simulink model "FwModelDirectWay"  (R2022b)
settings: Solver=FixedStepDiscrete  StartTime=0.0  StopTime=1  FixedStep=1e-6  RelTol=1e-3
values from neighbouring files (symbols this model uses):
  Ts = 0.0001    [Motor_PIParam_Get2.m]
undefined symbols (not defined in the file or in its folder): DiscIntNeverNeededParam, Motor_flux, Motor_Ld_Indctances, Motor_Lq_Indctances, Motor_Pn, Motor_Rs
libraries: powerlib_extras x2, spsGroundLib x1, spsPermanentMagnetSynchronousMachineLib x1, spsThreePhaseVIMeasurementLib x1, spsUniversalBridgeLib x1, spsDCVoltageSourceLib x1, spspowerguiLib x1
settings Model: DataDictionary=modelDictionary.sldd  Creator=yll  LastModifiedBy=yll

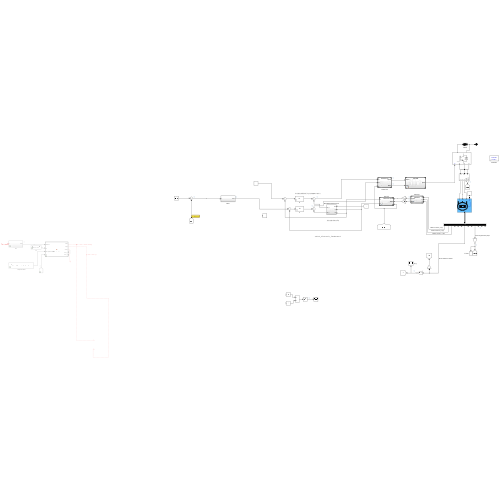
[thumbnail: Simulink's stored preview of the top-level diagram]
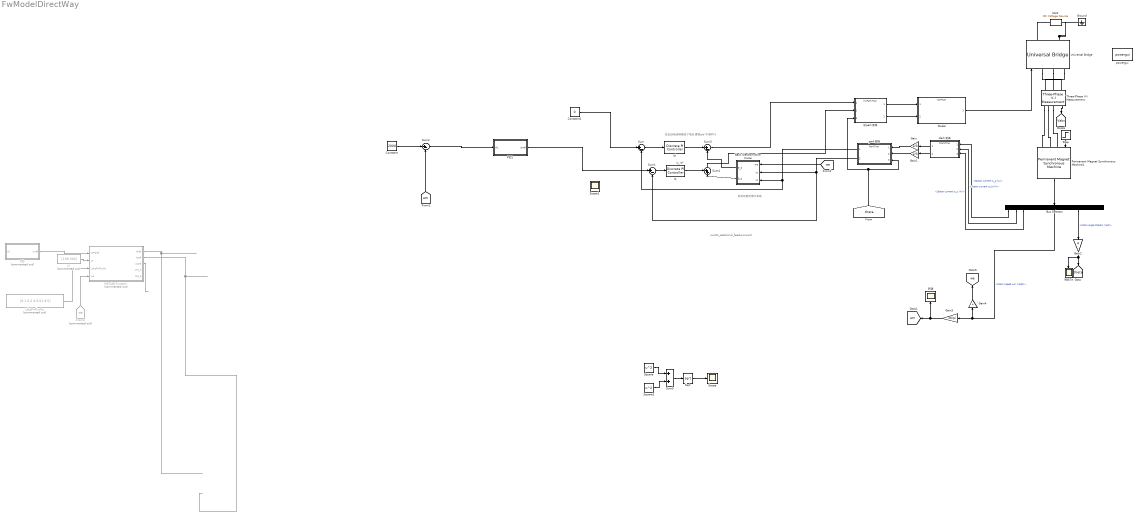
== system FwModelDirectWay ==
  note: switch_electronic_feedworward
  note: iq_ref
  note: 反电动势反馈子系统
  note: 在此处电流转换成了电压,要调pid 不调不行
  Back Electromotive Force : Subsystem
  Bus Selector : BusSelector  OutputSignals=Stator current is_a (A),Stator current is_b (A),Stator current is_c (A),Hall effect signal h_a,Hall effect signal h_b,Hall effect signal h_c,Rotor speed wm (rad/s),Stator current is_q (A),Stator current is_d (A),Rotor angle thetam (rad),Electromagnetic torque Te (N*m),Stator current is_q (A),Stator current is_d (A)
  Constant : Constant  Value=2000
  Constant1 : Constant  Value=0
  From3 : From  Commented=on  GotoTag=we  TagVisibility=global
  Gain : Gain  Gain=2/3
  Gain1 : Gain  Gain=2/3
  Gain2 : Gain  Gain=4
  Gain3 : Gain  Gain=30/pi
  Gain4 : Gain  Gain=4
  Ground : spsGroundLib/Ground  LConnTagsString=a
  Id : powerlib_extras/Discrete  Control Blocks/Discrete PI Controller  Kp=50  Ki=250  Par_Limits=[4000 -4000]  Init=0  Ts=1e-6
  Iq : powerlib_extras/Discrete  Control Blocks/Discrete PI Controller  Kp=50  Ki=250  Par_Limits=[4000 -4000]  Init=0  Ts=1e-6
  LdLqPnFluxRs : Constant  Commented=on  Value=[0.1 0.2 4 0.01 9.5]
  MATLAB Function : MATLAB Function  Commented=on  TreatAsAtomicUnit=on
  Model : ModelReference  ModelNameDialog=SVPWM.slx  SimulationMode=Normal  ModelReferenceVersion=1.6
  PID : Subsystem  Commented=on  VariantControl=true
  PID1 : Subsystem  VariantControl=true
  Permanent Magnet Synchronous Machine1 : spsPermanentMagnetSynchronousMachineLib/Permanent Magnet Synchronous Machine  NbPhases=3  FluxDistribution=Sinusoidal  RotorType=Salient-pole  MechanicalLoad=Torque Tm  PresetModel=No  ShowDetailedParameters=on  MeasurementBus=off  Resistance=Motor_Rs  Inductance=8.5e-3  dqInductances=[Motor_Ld_Indctances Motor_Lq_Indctances]  La=Motor_Ld_Indctances  MachineConstant=Flux linkage established by magnets (V.s)  Flux=Motor_flux  VoltageCst=145.1039  TorqueCst=1.2  Flat=120  Mechanical=[0.003 0 Motor_Pn 0]  PolePairs=2  InitialConditions=[0,0, 0,0]  InitialConditions5ph=[0 0 0 0 0 0]  RefAngle=Aligned with phase A axis (original Park)  IterativeDiscreteModel=Trapezoidal robust  TsBlock=-1  TsPowergui=0
  Scope : Scope
  Scope1 : Scope
  Sqrt : Sqrt
  Square : Math  Operator=square
  Square1 : Math  Operator=square
  Step : Step  Time=0.6  After=2  SampleTime=0
  Sum{,1..3} (4 alike) : Sum  Inputs=|+-
  Sum4 : Sum  Inputs=++|
  Sum5 : Sum
  Three-Phase V-I Measurement : spsThreePhaseVIMeasurementLib/Three-Phase V-I Measurement  VoltageMeasurement=phase-to-ground  SetLabelV=off  LabelV=Vabc  Vpu=off  VpuLL=off  CurrentMeasurement=yes  SetLabelI=off  LabelI=Iabc  Ipu=off  Pbase=100e6  Vbase=500e3  OutputType=Complex  PhasorSimulation=off  PSBequivalent=0
  UI : Constant  Commented=on  Value=[138 300]
  Universal Bridge : spsUniversalBridgeLib/Universal Bridge  Arms=3  SnubberResistance=1e3  SnubberCapacitance=inf  Device=IGBT / Diodes  Ron=1e-6  Lon=0  ForwardVoltages="[  0  0  ]"  ForwardVoltage="[  0  0  ]"  GTOparameters=[ 10e-6 , 20e-6 ]  IGBTparameters=[ 1e-6 , 2e-6 ]  Measurements=None  Measurements_2=None  converterType=Rectifier
  Vdc2 : spsDCVoltageSourceLib/DC Voltage Source  Amplitude=240  Measurements=None
  clark变换 : ModelReference  ModelNameDialog=ClarkTran.slx  SimulationMode=Normal  ModelReferenceVersion=1.13
  park变换 : ModelReference  ModelNameDialog=ParkTran.slx  SimulationMode=Normal  ModelReferenceVersion=1.9
  powergui : spspowerguiLib/powergui  Priority=1  SimulationMode=Discrete  SampleTime=1e-6  frequency=60  Iterations=50  frequencyindice=0  Pbase=100e6  ErrMax=1e-4  UnitsV=kV  UnitsW=MW  buscounter=0  FunctionMessages=off  echomessages=off  EnableUseOfTLC=off  CurrentSourceSwitches=off  DisableSnubberDevices=off  DisableRonSwitches=off  DisableVfSwitches=off  DisplayEquations=off  AutomaticDiscreteSolvers=off  SolverType=Tustin/Backward Euler (TBE)  Interpol=off  ExternalGateDelay=off  methode=off  Ts=10  x0status=blocks  SPID=off  SwTol=0  HookPort=off  NonlinearTolerance=1e-4  nMaxIteration=100  ContinueOnMaxIteration=off  RestoreLinks=warning  ResistiveCurrentMeasurement=off  Frange=[0:2:500]  Ylog=off  Xlog=on  ShowGrid=off  save=off  variable=ZData  structure=current_abc  ZoomFFT=off  StartTime=0.1  cycles=1  DisplayStyle=1  fundamental=1  FreqAxis=off  MaxFrequency=100  frequencyindicesteady=1  RmsSteady=1  display=off
  转矩Te : Scope
  转速 : Scope
  逆park变换 : ModelReference  ModelNameDialog=InvParkTran.slx  SimulationMode=Normal  ModelReferenceVersion=1.8
  tag scope: Vabc=global, theta=global, we=global, wm=global
  wires:
  Step/1 -> Permanent Magnet Synchronous Machine1/1
  Three-Phase V-I Measurement/1 -> [Vabc]
  Model/1 -> Universal Bridge/1
  Iq/1 -> Sum4/1
  Square1/1 -> Sum5/2
  clark变换/1 -> Gain/1
  Gain/1 -> park变换/1
  Back Electromotive Force/2(E_q) -> Sum4/2
  Square/1 -> Sum5/1
  [wm] -> Sum2/2
  Back Electromotive Force/1(E_d) -> Sum3/2
  Sum5/1 -> Sqrt/1
  [theta] -> 逆park变换/3, park变换/3
  clark变换/2 -> Gain1/1
  [we] -> Back Electromotive Force/1(we)
  park变换/1 -> Sum/2, Back Electromotive Force/3(id)
  Id/1 -> Sum3/1
  Sqrt/1 -> Scope/1
  Gain1/1 -> park变换/2
  Bus Selector/3 -> clark变换/3  "<Stator current is_c (A)>"
  逆park变换/2 -> Model/2
  Sum/1 -> Id/1
  Sum3/1 -> 逆park变换/1
  Sum4/1 -> 逆park变换/2
  逆park变换/1 -> Model/1
  park变换/2 -> Sum1/2, Back Electromotive Force/2(iq)
  Sum1/1 -> Iq/1
  Bus Selector/1 -> clark变换/1  "<Stator current is_a (A)>"
  Permanent Magnet Synchronous Machine1/1 -> Bus Selector/1
  Bus Selector/2 -> clark变换/2  "<Stator current is_b (A)>"
  Gain2/1 -> 转矩Te/1, [theta]
  Bus Selector/10 -> Gain2/1  "<Rotor angle thetam (rad)>"
  Gain4/1 -> [we]
  Gain3/1 -> [wm], 转速/1
  Bus Selector/7 -> Gain3/1, Gain4/1  "<Rotor speed wm (rad/s)>"
  Constant/1 -> Sum2/1
  From3/1 -> MATLAB Function/4(we)
  LdLqPnFluxRs/1 -> MATLAB Function/3(LdLqPnFluxRs)
  MATLAB Function/1(idref) -> ?
  UI/1 -> MATLAB Function/2(UI)
  PID/1(isref) -> MATLAB Function/1(isPidref)
  MATLAB Function/2(iqref) -> ?
  MATLAB Function/3(Zone) -> ?
  ? -> PID/1(In1)
  Sum2/1 -> PID1/1(In1)
  Constant1/1 -> Sum/1
  PID1/1(isref) -> Sum1/1
  connections:
  Universal Bridge/RConn2 -- Ground/LConn1 -- Vdc2/LConn1
  Vdc2/RConn1 -- Universal Bridge/RConn1
  Three-Phase V-I Measurement/RConn1 -- Permanent Magnet Synchronous Machine1/LConn1
  Three-Phase V-I Measurement/RConn3 -- Permanent Magnet Synchronous Machine1/LConn3
  Universal Bridge/LConn3 -- Three-Phase V-I Measurement/LConn3
  Three-Phase V-I Measurement/RConn2 -- Permanent Magnet Synchronous Machine1/LConn2
  Universal Bridge/LConn1 -- Three-Phase V-I Measurement/LConn1
  Universal Bridge/LConn2 -- Three-Phase V-I Measurement/LConn2

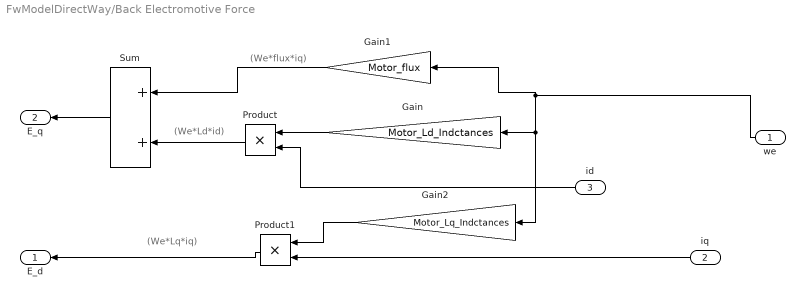
== system FwModelDirectWay/Back Electromotive Force ==
  note: (We*Lq*iq)
  note: (We*flux*iq)
  note: (We*Ld*id)
  we : Inport
  iq : Inport  Port=2
  id : Inport  Port=3
  Gain : Gain  Gain=Motor_Ld_Indctances
  Gain1 : Gain  Gain=Motor_flux
  Gain2 : Gain  Gain=Motor_Lq_Indctances
  Product : Product
  Product1 : Product
  Sum : Sum
  E_d : Outport
  E_q : Outport  Port=2
  wires:
  we/1 -> Gain2/1, Gain/1, Gain1/1
  Product1/1 -> E_d/1
  Gain1/1 -> Sum/1
  Sum/1 -> E_q/1
  Product/1 -> Sum/2
  id/1 -> Product/2
  iq/1 -> Product1/2
  Gain2/1 -> Product1/1
  Gain/1 -> Product/1

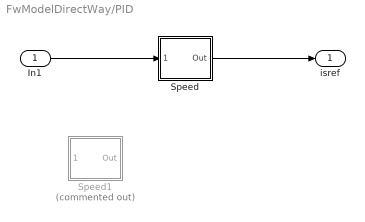
== system FwModelDirectWay/PID ==
  In1 : Inport
  Speed : Subsystem  AncestorBlock=|  DialogController=POWERSYS.PowerSysDialog  mask(Discrete PI Controller){Kpw=1, Kiw=1*50, Ba=0, Par_Limits=[3000 -3000], Init=0, Ts=1e-6}
      | powerlib_extras/Discrete 
      | Control Blocks/Discrete
      | PI Controller
      mask prompts: Kpw "Proportional gain (Kp):"; Kiw "Integral gain (Ki):"; Ba "feedback gain (Ba)"; Par_Limits "Output limits: [ Upper   Lower ]"; Init "Output initial value:"; Ts "Sample time:"
      mask help: This block implements a discrete PI controller.
      mask init:
      | UpperLimit=Par_Limits(1);
      | LowerLimit=Par_Limits(2);
      | power_initmask();
      settings: LibrarySourceBlock=|
      | powerlib_extras/Discrete
      | Control Blocks/Discrete
      | PI Controller
      mask Help: This block is part of a subset of blocks in the Extras library that does not have documentation associated with it, other than the block mask description.
      mask Display: disp('PI');
  Speed1 : Subsystem  Commented=on  AncestorBlock=|  DialogController=POWERSYS.PowerSysDialog  mask(Discrete PI Controller){Kpw=0.14, Kiw=0.14*50, Ba=0, Par_Limits=[800 -800], Init=0, Ts=Ts}
      | powerlib_extras/Discrete 
      | Control Blocks/Discrete
      | PI Controller
      mask prompts: Kpw "Proportional gain (Kp):"; Kiw "Integral gain (Ki):"; Ba "feedback gain (Ba)"; Par_Limits "Output limits: [ Upper   Lower ]"; Init "Output initial value:"; Ts "Sample time:"
      mask help: This block implements a discrete PI controller.
      mask init:
      | UpperLimit=Par_Limits(1);
      | LowerLimit=Par_Limits(2);
      | power_initmask();
      settings: LibrarySourceBlock=|
      | powerlib_extras/Discrete
      | Control Blocks/Discrete
      | PI Controller
      mask Help: This block is part of a subset of blocks in the Extras library that does not have documentation associated with it, other than the block mask description.
      mask Display: disp('PI');
  isref : Outport
  wires:
  Speed/1(Out) -> isref/1
  In1/1 -> Speed/1(Error)

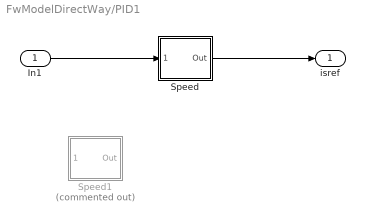
== system FwModelDirectWay/PID1 ==
  In1 : Inport
  Speed : Subsystem  AncestorBlock=|  DialogController=POWERSYS.PowerSysDialog  mask(Discrete PI Controller){Kpw=0.14, Kiw=0.14*50, Ba=0, Par_Limits=[6000 -6000], Init=0, Ts=1e-6}
      | powerlib_extras/Discrete 
      | Control Blocks/Discrete
      | PI Controller
      mask prompts: Kpw "Proportional gain (Kp):"; Kiw "Integral gain (Ki):"; Ba "feedback gain (Ba)"; Par_Limits "Output limits: [ Upper   Lower ]"; Init "Output initial value:"; Ts "Sample time:"
      mask help: This block implements a discrete PI controller.
      mask init:
      | UpperLimit=Par_Limits(1);
      | LowerLimit=Par_Limits(2);
      | power_initmask();
      settings: LibrarySourceBlock=|
      | powerlib_extras/Discrete
      | Control Blocks/Discrete
      | PI Controller
      mask Help: This block is part of a subset of blocks in the Extras library that does not have documentation associated with it, other than the block mask description.
      mask Display: disp('PI');
  Speed1 : Subsystem  Commented=on  AncestorBlock=|  DialogController=POWERSYS.PowerSysDialog  mask(Discrete PI Controller){Kpw=0.14, Kiw=0.14*50, Ba=0, Par_Limits=[800 -800], Init=0, Ts=Ts}
      | powerlib_extras/Discrete 
      | Control Blocks/Discrete
      | PI Controller
      mask prompts: Kpw "Proportional gain (Kp):"; Kiw "Integral gain (Ki):"; Ba "feedback gain (Ba)"; Par_Limits "Output limits: [ Upper   Lower ]"; Init "Output initial value:"; Ts "Sample time:"
      mask help: This block implements a discrete PI controller.
      mask init:
      | UpperLimit=Par_Limits(1);
      | LowerLimit=Par_Limits(2);
      | power_initmask();
      settings: LibrarySourceBlock=|
      | powerlib_extras/Discrete
      | Control Blocks/Discrete
      | PI Controller
      mask Help: This block is part of a subset of blocks in the Extras library that does not have documentation associated with it, other than the block mask description.
      mask Display: disp('PI');
  isref : Outport
  wires:
  Speed/1(Out) -> isref/1
  In1/1 -> Speed/1(Error)

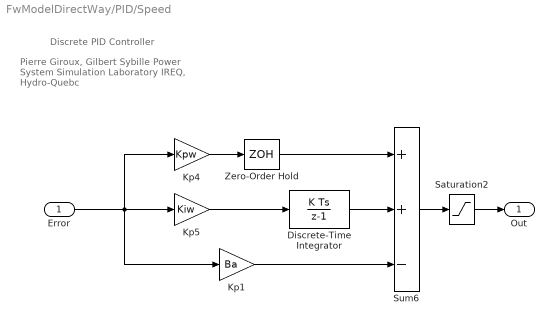
== system FwModelDirectWay/PID/Speed ==
  note: Pierre Giroux, Gilbert Sybille
      | Power System Simulation Laboratory
      | IREQ, Hydro-Quebc
  note: Discrete PID Controller
  Error : Inport  SampleTime=Ts
  Discrete-Time Integrator : DiscreteIntegrator  InitialCondition=Init  SampleTime=Ts  LimitOutput=on  UpperSaturationLimit=UpperLimit  LowerSaturationLimit=LowerLimit  ICPrevOutput=DiscIntNeverNeededParam  ICPrevScaledInput=DiscIntNeverNeededParam
  Kp1 : Gain  Gain=Ba  SaturateOnIntegerOverflow=on  SampleTime=Ts  OutDataTypeStr=Inherit: Same as input  ParamDataTypeStr=Inherit: Same as input
  Kp4 : Gain  Gain=Kpw  SaturateOnIntegerOverflow=on  SampleTime=Ts  OutDataTypeStr=Inherit: Same as input  ParamDataTypeStr=Inherit: Same as input
  Kp5 : Gain  Gain=Kiw  SaturateOnIntegerOverflow=on  SampleTime=Ts  OutDataTypeStr=Inherit: Same as input  ParamDataTypeStr=Inherit: Same as input
  Saturation2 : Saturate  UpperLimit=UpperLimit  LowerLimit=LowerLimit  SampleTime=Ts
  Sum6 : Sum  Inputs=++-  InputSameDT=on  SaturateOnIntegerOverflow=on  SampleTime=Ts  OutDataTypeStr=Inherit: Same as first input
  Zero-Order Hold : ZeroOrderHold  SampleTime=Ts
  Out : Outport  SampleTime=Ts  InitialOutput=0
  wires:
  Kp1/1 -> Sum6/3
  Sum6/1 -> Saturation2/1
  Kp5/1 -> Discrete-Time Integrator/1
  Kp4/1 -> Zero-Order Hold/1
  Discrete-Time Integrator/1 -> Sum6/2
  Saturation2/1 -> Out/1
  Zero-Order Hold/1 -> Sum6/1
  Error/1 -> Kp4/1, Kp5/1, Kp1/1

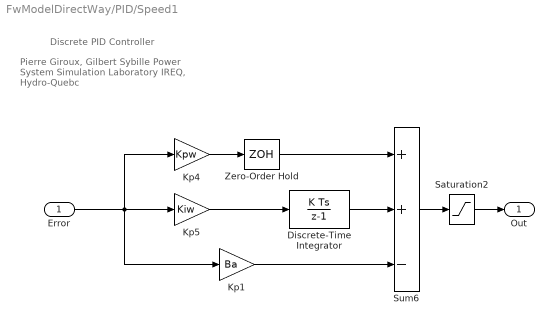
== system FwModelDirectWay/PID/Speed1 ==
  note: Discrete PID Controller
  note: Pierre Giroux, Gilbert Sybille
      | Power System Simulation Laboratory
      | IREQ, Hydro-Quebc
  Error : Inport  SampleTime=Ts
  Discrete-Time Integrator : DiscreteIntegrator  InitialCondition=Init  SampleTime=Ts  LimitOutput=on  UpperSaturationLimit=UpperLimit  LowerSaturationLimit=LowerLimit  ICPrevOutput=DiscIntNeverNeededParam  ICPrevScaledInput=DiscIntNeverNeededParam
  Kp1 : Gain  Gain=Ba  SaturateOnIntegerOverflow=on  SampleTime=Ts  OutDataTypeStr=Inherit: Same as input  ParamDataTypeStr=Inherit: Same as input
  Kp4 : Gain  Gain=Kpw  SaturateOnIntegerOverflow=on  SampleTime=Ts  OutDataTypeStr=Inherit: Same as input  ParamDataTypeStr=Inherit: Same as input
  Kp5 : Gain  Gain=Kiw  SaturateOnIntegerOverflow=on  SampleTime=Ts  OutDataTypeStr=Inherit: Same as input  ParamDataTypeStr=Inherit: Same as input
  Saturation2 : Saturate  UpperLimit=UpperLimit  LowerLimit=LowerLimit  SampleTime=Ts
  Sum6 : Sum  Inputs=++-  InputSameDT=on  SaturateOnIntegerOverflow=on  SampleTime=Ts  OutDataTypeStr=Inherit: Same as first input
  Zero-Order Hold : ZeroOrderHold  SampleTime=Ts
  Out : Outport  SampleTime=Ts  InitialOutput=0
  wires:
  Error/1 -> Kp1/1, Kp5/1, Kp4/1
  Zero-Order Hold/1 -> Sum6/1
  Saturation2/1 -> Out/1
  Discrete-Time Integrator/1 -> Sum6/2
  Kp4/1 -> Zero-Order Hold/1
  Kp5/1 -> Discrete-Time Integrator/1
  Sum6/1 -> Saturation2/1
  Kp1/1 -> Sum6/3

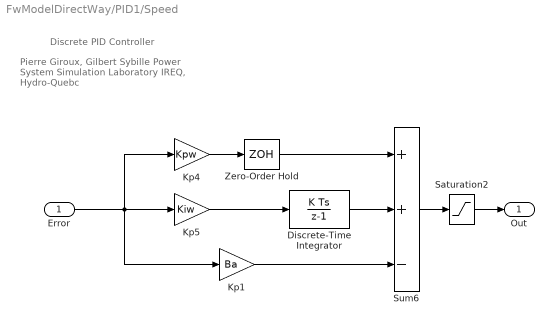
== system FwModelDirectWay/PID1/Speed ==
  note: Pierre Giroux, Gilbert Sybille
      | Power System Simulation Laboratory
      | IREQ, Hydro-Quebc
  note: Discrete PID Controller
  Error : Inport  SampleTime=Ts
  Discrete-Time Integrator : DiscreteIntegrator  InitialCondition=Init  SampleTime=Ts  LimitOutput=on  UpperSaturationLimit=UpperLimit  LowerSaturationLimit=LowerLimit  ICPrevOutput=DiscIntNeverNeededParam  ICPrevScaledInput=DiscIntNeverNeededParam
  Kp1 : Gain  Gain=Ba  SaturateOnIntegerOverflow=on  SampleTime=Ts  OutDataTypeStr=Inherit: Same as input  ParamDataTypeStr=Inherit: Same as input
  Kp4 : Gain  Gain=Kpw  SaturateOnIntegerOverflow=on  SampleTime=Ts  OutDataTypeStr=Inherit: Same as input  ParamDataTypeStr=Inherit: Same as input
  Kp5 : Gain  Gain=Kiw  SaturateOnIntegerOverflow=on  SampleTime=Ts  OutDataTypeStr=Inherit: Same as input  ParamDataTypeStr=Inherit: Same as input
  Saturation2 : Saturate  UpperLimit=UpperLimit  LowerLimit=LowerLimit  SampleTime=Ts
  Sum6 : Sum  Inputs=++-  InputSameDT=on  SaturateOnIntegerOverflow=on  SampleTime=Ts  OutDataTypeStr=Inherit: Same as first input
  Zero-Order Hold : ZeroOrderHold  SampleTime=Ts
  Out : Outport  SampleTime=Ts  InitialOutput=0
  wires:
  Kp1/1 -> Sum6/3
  Sum6/1 -> Saturation2/1
  Kp5/1 -> Discrete-Time Integrator/1
  Kp4/1 -> Zero-Order Hold/1
  Discrete-Time Integrator/1 -> Sum6/2
  Saturation2/1 -> Out/1
  Zero-Order Hold/1 -> Sum6/1
  Error/1 -> Kp4/1, Kp5/1, Kp1/1

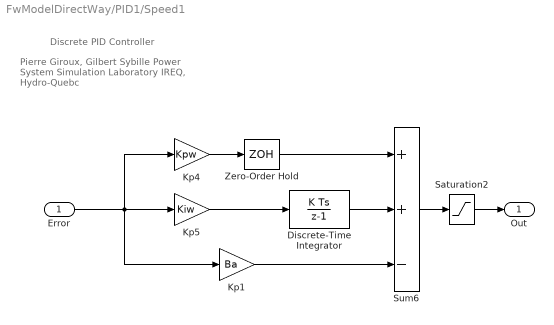
== system FwModelDirectWay/PID1/Speed1 ==
  note: Discrete PID Controller
  note: Pierre Giroux, Gilbert Sybille
      | Power System Simulation Laboratory
      | IREQ, Hydro-Quebc
  Error : Inport  SampleTime=Ts
  Discrete-Time Integrator : DiscreteIntegrator  InitialCondition=Init  SampleTime=Ts  LimitOutput=on  UpperSaturationLimit=UpperLimit  LowerSaturationLimit=LowerLimit  ICPrevOutput=DiscIntNeverNeededParam  ICPrevScaledInput=DiscIntNeverNeededParam
  Kp1 : Gain  Gain=Ba  SaturateOnIntegerOverflow=on  SampleTime=Ts  OutDataTypeStr=Inherit: Same as input  ParamDataTypeStr=Inherit: Same as input
  Kp4 : Gain  Gain=Kpw  SaturateOnIntegerOverflow=on  SampleTime=Ts  OutDataTypeStr=Inherit: Same as input  ParamDataTypeStr=Inherit: Same as input
  Kp5 : Gain  Gain=Kiw  SaturateOnIntegerOverflow=on  SampleTime=Ts  OutDataTypeStr=Inherit: Same as input  ParamDataTypeStr=Inherit: Same as input
  Saturation2 : Saturate  UpperLimit=UpperLimit  LowerLimit=LowerLimit  SampleTime=Ts
  Sum6 : Sum  Inputs=++-  InputSameDT=on  SaturateOnIntegerOverflow=on  SampleTime=Ts  OutDataTypeStr=Inherit: Same as first input
  Zero-Order Hold : ZeroOrderHold  SampleTime=Ts
  Out : Outport  SampleTime=Ts  InitialOutput=0
  wires:
  Error/1 -> Kp1/1, Kp5/1, Kp4/1
  Zero-Order Hold/1 -> Sum6/1
  Saturation2/1 -> Out/1
  Discrete-Time Integrator/1 -> Sum6/2
  Kp4/1 -> Zero-Order Hold/1
  Kp5/1 -> Discrete-Time Integrator/1
  Sum6/1 -> Saturation2/1
  Kp1/1 -> Sum6/3

== matlab function FwModelDirectWay/MATLAB Function ==
  data: isPidref input; idref output; UI input; LdLqPnFluxRs input; we input; iqref output; Zone output; We_b output; We_a output
% 基于直接计算法的弱磁控制
% 参数：
% isPidref 经过pid 调节后的定子电流 UI 最大电压和最大电流
% LdLqPnFluxRs d轴电感 q轴电感 极对数 磁链 定子电阻
% 返回值:
% 输出idref iqref 为输出的id iq电流 Zone 为当前所采取的控制  

function [idref, iqref,Zone,We_b,We_a] =FW_Direct(isPidref, UI, LdLqPnFluxRs,we)

%%%%%%%%%%%%%%%%%%%%%%%%%%%%%%%%%%%%%
%               读取数据             % 
Udc=UI(1);
I=UI(2);
Ld=LdLqPnFluxRs(1);
Lq=LdLqPnFluxRs(2);
pn=LdLqPnFluxRs(3);%转子对数
flux=LdLqPnFluxRs(4);%永磁体磁链
Rs=LdLqPnFluxRs(5); %定子电阻
Zone=0;


Umax=Udc*2/pi; %最大电压限制
Imax=I*sqrt(2);% 最大电流限制
%%%%%%%%%%%%%%%%%%%%%%%%%%%%%%%%%%%%%
%        计算过渡转速 We_a 与 We_b   %
IdA=(-flux+sqrt(flux^2+8*(Ld-Lq)^2*Imax^2))/(4*(Ld-Lq));
IqA=sqrt(Imax^2 - IdA^2);
We_a=sqrt(Umax^2/((Ld*IdA+flux)^2+(Lq*IqA)^2));

tempB_a=-flux*Ld*(2*Ld-Lq);
tempB_b=2*(Ld^2+Lq^2)*(Ld-Lq);
tempB_c=Ld^2*(2*Ld-Lq)^2-4*Ld*(Ld-Lq)*(Ld^2+Lq^2);
tempB_d=Lq^2*(Ld-Lq)^2*(Ld^2+Lq^2);
tempB_e=sqrt(tempB_c*flux^2+4*Imax^2*tempB_d);
IdB=tempB_a+tempB_e/tempB_b;
IqB=sqrt(Imax^2-IdB^2);
We_b=sqrt(Umax^2/((Ld*IdB+flux)^2+(Lq*IqB)^2));


%%%%%%%%%%%%%%%%%%%%%%%%%%%%%%%%%%%%%

if(we<=We_a)
    if(isPidref<IqA) 
        % MPTA控制
        iqref = isPidref; 
        idref=-flux+sqrt(flux^2+4*(Ld-Lq)^2*iqref^2)/(2*(Ld-Lq)); 
        Zone=0;
    else
        % 此时已达最大
        iqref=IqA;
        idref=IdA;
        Zone=1;
    end
else
    if(we<We_b)
        %FW
        idAB =(-flux*Ld+sqrt(flux^2*Ld^2-(Ld^2-Lq^2)*(flux^2+Lq^2*Imax^2-(Umax/we)^2)))/(Ld^2-Lq^2);
        iqAB =sqrt(Imax^2 - idAB^2);
        if(isPidref<iqAB)
            idref=(-flux*Ld+sqrt(flux^2*Ld^2-(Ld^2-Lq^2)*(flux^2+Lq^2*isPidref^2-(Umax/we)^2)))/(Ld^2-Lq^2);
            iqref=isPidref;
            Zone=2;
        else
            idref=idAB;
            iqref=iqAB;
            Zone=3;
        end
    else
        idMTPV=-flux/Ld+(-flux*Lq+sqrt(flux^2*Lq^2+8*(Ld-Lq)^2*(Umax/we)^2))/(4*Ld*(Ld-Lq));
        iqMTPV=sqrt((Umax^2/we^2 - (Ld*idMTPV*flux)^2)/Lq^2); 
        if(isPidref<iqMTPV)
            iqref=isPidref;             
            idref=-flux/Ld+(-flux*Lq+Lq*sqrt(flux^2+4*(Ld-Lq)^2*iqref^2))/(2*Ld*(Ld-Lq));
            Zone=5;
        else
            idref=idMTPV;
            iqref=iqMTPV;
            Zone=4;
        end
    end
end
